simulink model "HBC_PHY_Layer"  (R2024a)
settings: Solver=FixedStepDiscrete  StartTime=0.0  StopTime=5E-2  RelTol=1e-3
values from neighbouring files (symbols this model uses):
  cfg = HBC_PHYFrameConfig(DataRate = '328Kbps', PilotInfo = '128', PSDULength = 254)    [MonteCarloSimulations.m]
libraries: hdlsllib x10, whdlio x1, commhdlcrc x1, commseqgen3 x1, vivadosimlib x1
settings Model: Creator=sookn  LastModifiedBy=sookn
settings OptimizationCC: BlockReduction=off  ConditionallyExecuteInputs=off  DefaultParameterBehavior=Inlined  OptimizeBlockIOStorage=off  EnhancedBackFolding=on  PassReuseOutputArgsAs=Individual arguments  OptimizeBlockOrder=speed  DifferentSizesBufferReuse=on  EfficientTunableParamExpr=on
settings DebuggingCC: SingleTaskRateTransMsg=error  ParameterTunabilityLossMsg=error
settings HardwareCC: ProdBitPerPointer=32  ProdBitPerSizeT=32  ProdBitPerPtrDiffT=32  ProdLargestAtomicFloat=None  ProdIntDivRoundTo=Undefined  ProdEndianess=Unspecified  ProdWordSize=32  ProdHWDeviceType=ASIC/FPGA->ASIC/FPGA  TargetBitPerPointer=64  TargetBitPerSizeT=64  TargetBitPerPtrDiffT=64  TargetLongLongMode=on  TargetIntDivRoundTo=Zero  TargetEndianess=LittleEndian  TargetWordSize=64  TargetHWDeviceType=Generic->Custom  ProdEqTarget=off
settings SFSimCC: MATLABDynamicMemAlloc=off
settings RTWCC: Description=SystemVerilog DPI Component Generator  SystemTargetFile=systemverilog_dpi_ert.tlc  TemplateMakefile=systemverilog_dpi_ert_default_tmf
settings CodeAppCC: ForceParamTrailComments=on  IgnoreCustomStorageClasses=off  MaxIdLength=256  OperatorAnnotations=on  SimulinkDataObjDesc=on  SFDataObjDesc=on  InsertBlockDesc=on
settings DPIERTTargetCC: TargetFcnLib=ansi_tfl_table_tmw.mat  GenFloatMathFcnCalls=NOT IN USE  TargetLangStandard=C99 (ISO)  CodeReplacementLibrary=None  UtilityFuncGeneration=Auto  MultiwordTypeDef=System defined  MultiwordLength=2048  DynamicStringBufferSize=256  GenerateFullHeader=on  InferredTypesCompatibility=off  GenerateSampleERTMain=off  GenerateTestInterfaces=off  ModelReferenceCompliant=on  ParMdlRefBuildCompliant=on  CompOptLevelCompliant=off  ConcurrentExecutionCompliant=off  IncludeMdlTerminateFcn=on  CombineOutputUpdateFcns=off  CombineSignalStateStructs=on  GroupInternalDataByFunction=off  SuppressErrorStatus=off  IncludeFileDelimiter=Auto  ERTCustomFileBanners=on  SupportAbsoluteTime=on  LogVarNameModifier=rt_  MatFileLogging=off  CodeInterfacePackaging=Reusable function  PurelyIntegerCode=off  SupportNonFinite=on  SupportComplex=on  SupportContinuousTime=on  SupportNonInlinedSFcns=on  RemoveDisableFunc=off  RemoveResetFunc=on  SupportVariableSizeSignals=off  ParenthesesLevel=Nominal  CastingMode=Nominal  MATLABClassNameForMDSCustomization=Simulink.SoftwareTarget.TargetSpecificTriggerConfigurationBase  ModelStepFunctionPrototypeControlCompliant=on  CPPClassGenCompliant=off  AutosarCompliant=off  MDXCompliant=off  GRTInterface=off  GenerateAllocFcn=on  UseToolchainInfoCompliant=on  GenerateSharedConstants=on  CoderGroups=[]  AccessMethods=[]  LookupTableObjectStructAxisOrder=1,2,3,4,...  LUTObjectStructOrderExplicitValues=Size,Breakpoints,Table  LUTObjectStructOrderEvenSpacing=Size,Breakpoints,Table  ArrayLayout=Column-major  UnsupportedSFcnMsg=error  ERTHeaderFileRootName=$R$E  ERTSourceFileRootName=$R$E  ERTDataFileRootName=$R_data  InstructionSetFMA=off  OptimizeReductions=off  LogToMDFFile=off  GenerateASAP2=off  DSAsUniqueAccess=off  ExtMode=off  ExtModeTransport=0  ExtModeStaticAlloc=off  ExtModeAutomaticAllocSize=on  ExtModeMaxTrigDuration=10  ExtModeStaticAllocSize=1000000  ExtModeTesting=off  ExtModeMexFile=ext_comm  ExtModeIntrfLevel=Level1  InlinedParameterPlacement=NonHierarchical  TargetOS=BareBoardExample  MultiInstanceErrorCode=Error  RootIOFormat=Part of model data structure  RTWCAPISignals=on  RTWCAPIParams=off  RTWCAPIStates=off  RTWCAPIRootIO=off  ERTSrcFileBannerTemplate=ert_code_template.cgt  ERTHdrFileBannerTemplate=ert_code_template.cgt  ERTDataSrcFileTemplate=ert_code_template.cgt  ERTDataHdrFileTemplate=ert_code_template.cgt  ERTCustomFileTemplate=example_file_process.tlc  EnableDataOwnership=off  SignalDisplayLevel=10  ParamTuneLevel=10  GlobalDataDefinition=Auto  DataDefinitionFile=global.c  GlobalDataReference=Auto  ERTFilePackagingFormat=Modular  RateTransitionBlockCode=Inline  DataReferenceFile=global.h  PreserveExpressionOrder=off  PreserveIfCondition=off  ConvertIfToSwitch=on  PreserveExternInFcnDecls=on  PreserveStaticInFcnDecls=on  SuppressUnreachableDefaultCases=on  EnableSignedLeftShifts=on  EnableSignedRightShifts=on  ImplementImageWithCVMat=off  IndentStyle=K&R  IndentSize=2  NewlineStyle=Default  MaxLineWidth=80  EnableUserReplacementTypes=off  MaxIdInt64=MAX_int64_T  MinIdInt64=MIN_int64_T  MaxIdUint64=MAX_uint64_T  MaxIdInt32=MAX_int32_T  MinIdInt32=MIN_int32_T  MaxIdUint32=MAX_uint32_T  MaxIdInt16=MAX_int16_T  MinIdInt16=MIN_int16_T  MaxIdUint16=MAX_uint16_T  MaxIdInt8=MAX_int8_T  MinIdInt8=MIN_int8_T  MaxIdUint8=MAX_uint8_T  BooleanTrueId=true  BooleanFalseId=false  MemSecPackage=--- None ---  MemSecDataConstants=Default  MemSecDataIO=Default  MemSecDataInternal=Default  MemSecDataParameters=Default  MemSecFuncInitTerm=Default  MemSecFuncExecute=Default  MemSecFuncSharedUtil=Default  GroupConstants=Default  GroupRootInputs=Default  GroupRootOutputs=Default  GroupInternal=Default  GroupParameters=Default  GroupDataTransfer=Default  GroupSharedLocalDataStores=Default  GroupInstanceSpecificParameters=Default  GroupModelData=Default  ArrayContainerType=C-style array  DPICustomizeSystemVerilogCode=off  DPISystemVerilogTemplate=svdpi_event.vgt  DPIReportRunTimeError=off  DPIScalarizePorts=off  DPIRunTimeErrorSeverity=Fatal  DPIGenerateTestBench=off  DPITestBenchSimulator=Mentor Graphics Questasim  DPITestPointAccessFcnInterface=None  DPIFixedPointDataType=CompatibleCType  DPIPortConnection=Port list  DPICompositeDataType=Flattened  DPIComponentTemplateType=Sequential

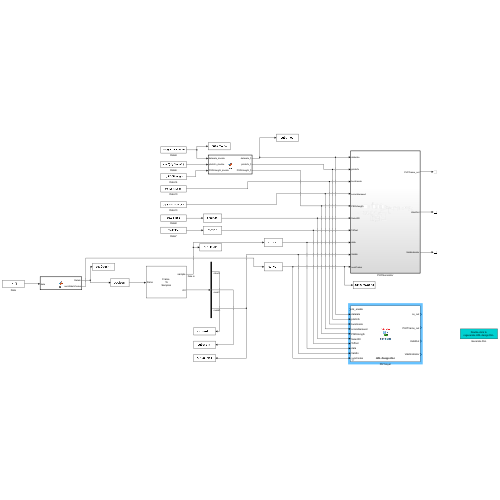
[thumbnail: Simulink's stored preview of the top-level diagram]
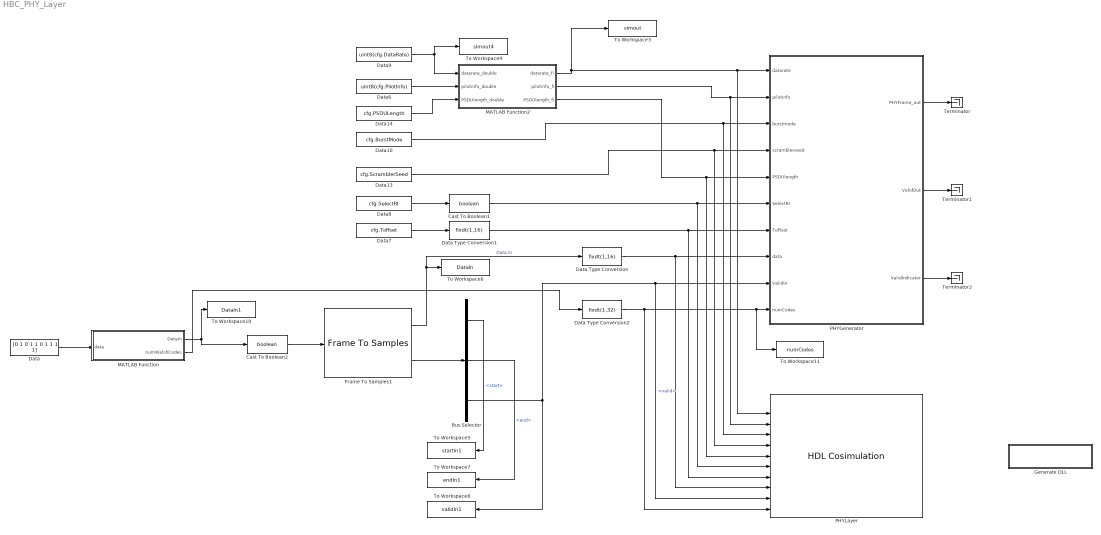
== system HBC_PHY_Layer ==
  Bus Selector : BusSelector  OutputSignals=start,end,valid
  Cast To Boolean1 : DataTypeConversion  OutDataTypeStr=boolean  SaturateOnIntegerOverflow=off  RndMeth=Floor
  Cast To Boolean2 : DataTypeConversion  OutDataTypeStr=boolean  SaturateOnIntegerOverflow=off  RndMeth=Floor
  Data : Constant  Value=[0 1 0 1 1 0 1 1 1 1]  SampleTime=-1
  Data Type Conversion : DataTypeConversion  OutMax=[1]  OutDataTypeStr=fixdt(1,16)  SaturateOnIntegerOverflow=off  RndMeth=Floor
  Data Type Conversion1 : DataTypeConversion  OutMax=[16]  OutDataTypeStr=fixdt(1,16)  SaturateOnIntegerOverflow=off  RndMeth=Floor
  Data Type Conversion2 : DataTypeConversion  OutMax=[32]  OutDataTypeStr=fixdt(1,32)  SaturateOnIntegerOverflow=off  RndMeth=Floor
  Data10 : Constant  Value=cfg.BurstMode  SampleTime=(9056*8)/(42E6)
  Data13 : Constant  Value=cfg.ScramblerSeed  SampleTime=(9056*8)/(42E6)
  Data14 : Constant  Value=cfg.PSDULength  SampleTime=-1
  Data6 : Constant  Value=uint8(cfg.PilotInfo)  SampleTime=-1
  Data7 : Constant  Value=cfg.Toffset  SampleTime=(9056*8)/(42E6)
  Data8 : Constant  Value=cfg.SelectRI  SampleTime=(9056*8)/(42E6)
  Data9 : Constant  Value=uint8(cfg.DataRate)  SampleTime=-1
  Frame To Samples1 : whdlio/Frame To Samples  InterSampleIdleCycles=0  InterFrameIdleCycles=4  OutputSize=1  InterleaveSamples=off
  Generate DLL : Subsystem
      settings: OpenFcn=eval('hdlverifier_gendll_PHYLayer');
      mask Display: disp(['Double-click to' char(10) 'regenerate HDL design DLL'])
  MATLAB Function : MATLAB Function  TreatAsAtomicUnit=on
  MATLAB Function2 : MATLAB Function  TreatAsAtomicUnit=on
  PHYGenerator : Subsystem  TreatAsAtomicUnit=on
  PHYLayer : vivadosimlib/HDL Cosimulation  PortPaths=/PHYLayer/clk_enable;/PHYLayer/datarate;/PHYLayer/pilotinfo;/PHYLayer/burstmode;/PHYLayer/scramblerseed;/PHYLayer/PSDUlength;/PHYLayer/SelectRI;/PHYLayer/Toffset;/PHYLayer/data;/PHYLayer/ValidIn;/PHYLayer/numCodes;/PHYLayer/ce_out;/PHYLayer/PHYFrame_out;/PHYLayer/ValidOut;/PHYLayer/ValidIndicator;  PortModes=[1 1 1 1 1 1 1 1 1 1 1 2 2 2 2 ]  PortTimes=[-1,-1,-1,-1,-1,-1,-1,-1,-1,-1,-1,1,1,1,1]  PortSigns=[-1,-1,-1,-1,-1,-1,-1,-1,-1,-1,-1,-1,-1,-1,-1,]  PortFracLengths=[0,0,0,0,0,0,0,0,0,0,0,0,0,0,0]  PortWordLengths=[-1,-1,-1,-1,-1,-1,-1,-1,-1,-1,-1,1,1,1,1]  PortHDLWordSizes=[1,3,3,1,1,9,1,16,16,1,32,1,1,1,1]  CommLocal=on  CommSharedMemory=off  CommPortNumber=0  CommShowInfo=on  ClockPaths=/PHYLayer/clk;/PHYLayer/reset;  ClockModes=[2 3 ]  ClockTimes=[1e-08 8e-09 ]  TimingMode=s  TimingScaleFactor=1  idxCellArray={'UNUSED_VAR'}  CosimBypass=Full Simulation  AllowDirectFeedthrough=on  ProductName=EDA Simulator Link VS  RunAutoTimescale=on  HdlClocks=/PHYLayer/clk 10 ns;  PreRunTime=10  PreRunTimeUnit=ns
  Terminator : Terminator
  Terminator1 : Terminator
  Terminator2 : Terminator
  To Workspace10 : ToWorkspace  VariableName=DataIn1  SaveFormat=Structure With Time  SampleTime=-1
  To Workspace11 : ToWorkspace  VariableName=numCodes  SaveFormat=Structure With Time  SampleTime=-1
  To Workspace3 : ToWorkspace  VariableName=simout  SaveFormat=Structure With Time  SampleTime=-1
  To Workspace4 : ToWorkspace  VariableName=simout4  SaveFormat=Structure With Time  SampleTime=-1
  To Workspace5 : ToWorkspace  VariableName=startIn1  SaveFormat=Structure With Time  SampleTime=-1
  To Workspace6 : ToWorkspace  VariableName=DataIn  SaveFormat=Structure With Time  SampleTime=-1
  To Workspace7 : ToWorkspace  VariableName=endIn1  SaveFormat=Structure With Time  SampleTime=-1
  To Workspace8 : ToWorkspace  VariableName=validIn1  SaveFormat=Structure With Time  SampleTime=-1
  wires:
  Cast To Boolean2/1 -> Frame To Samples1/1
  Data9/1 -> MATLAB Function2/1(datarate_double), To Workspace4/1
  Data14/1 -> MATLAB Function2/3(PSDUlength_double)
  Frame To Samples1/1 -> Data Type Conversion/1, To Workspace6/1  "Data In"
  Data13/1 -> PHYLayer/5, PHYGenerator/4(scramblerseed)
  Data8/1 -> Cast To Boolean1/1
  Data Type Conversion1/1 -> PHYLayer/8, PHYGenerator/7(Toffset)
  MATLAB Function2/2(pilotinfo_fi) -> PHYLayer/3, PHYGenerator/2(pilotinfo)
  MATLAB Function/2(numWalshCodes) -> Data Type Conversion2/1
  Frame To Samples1/2 -> Bus Selector/1
  Data Type Conversion2/1 -> PHYLayer/11, To Workspace11/1, PHYGenerator/10(numCodes)
  Data6/1 -> MATLAB Function2/2(pilotinfo_double)
  Bus Selector/3 -> PHYLayer/10, PHYGenerator/9(ValidIn), To Workspace8/1  "<valid>"
  MATLAB Function2/3(PSDUlength_fi) -> PHYLayer/6, PHYGenerator/5(PSDUlength)
  PHYGenerator/1(PHYFrame_out) -> Terminator/1
  Bus Selector/2 -> To Workspace7/1  "<end>"
  MATLAB Function/1(DataIn) -> Cast To Boolean2/1, To Workspace10/1
  PHYGenerator/2(ValidOut) -> Terminator1/1
  Cast To Boolean1/1 -> PHYLayer/7, PHYGenerator/6(SelectRI)
  Bus Selector/1 -> To Workspace5/1  "<start>"
  Data/1 -> MATLAB Function/1(data)
  Data7/1 -> Data Type Conversion1/1
  MATLAB Function2/1(datarate_fi) -> To Workspace3/1, PHYLayer/2, PHYGenerator/1(datarate)
  Data10/1 -> PHYLayer/4, PHYGenerator/3(burstmode)
  PHYGenerator/3(ValidIndicator) -> Terminator2/1
  Data Type Conversion/1 -> PHYLayer/9, PHYGenerator/8(data)

== system HBC_PHY_Layer/Generate DLL ==

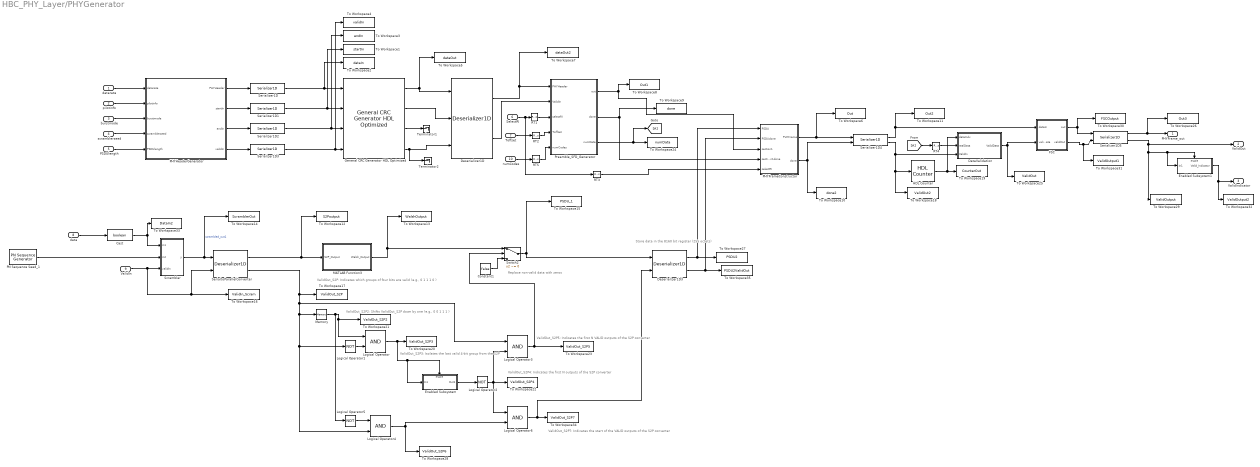
== system HBC_PHY_Layer/PHYGenerator ==
  note: Replace non-valid data with zeros
  note: ValidOut_S2P: Indicates which groups of four bits are valid (e.g., 0 1 1 1 0 )
  note: ValidOut_S2P2: Shifts ValidOut_S2P down by one (e.g., 0 0 1 1 1 )
  note: ValidOut_S2P3: Isolates the last valid 4-bit group from the S2P
  note: ValidOut_S2P4: Indicates the first N outputs of the S2P converter
  note: ValidOut_S2P5: Indicates the first N VALID outputs of the S2P converter
  note: ValidOut_S2P7: Indicates the start of the VALID outputs of the S2P converter
  note: Store data in the 8160 bit register (255 octets)
  datarate : Inport
  pilotinfo : Inport  Port=2
  burstmode : Inport  Port=3
  scramblerseed : Inport  Port=4
  PSDUlength : Inport  Port=5
  SelectRI : Inport  Port=6
  Toffset : Inport  Port=7
  data : Inport  Port=8
  ValidIn : Inport  Port=9
  numCodes : Inport  Port=10
  Cast : DataTypeConversion  OutDataTypeStr=boolean  SaturateOnIntegerOverflow=off  RndMeth=Floor
  Constant1 : Constant  Value=false  SampleTime=-1
  DataValidation : MATLAB Function  TreatAsAtomicUnit=on
  Deserializer1D : hdlsllib/HDL Operations/Deserializer1D  Ratio=4  IdleCycles=0  InitialCondition=0  startIn=on  validIn=on  validOut=on  inputDataDimensions=-1  inputSampleTime=-1  inputSignalType=auto
  Deserializer1D3 : hdlsllib/HDL Operations/Deserializer1D  Ratio=510  IdleCycles=0  InitialCondition=0  startIn=on  validIn=off  validOut=on  inputDataDimensions=-1  inputSampleTime=-1  inputSignalType=auto
  Enabled Subsystem : Subsystem  TreatAsAtomicUnit=on
  Enabled Subsystem1 : Subsystem  TreatAsAtomicUnit=on
  FSC : MATLAB Function  TreatAsAtomicUnit=on
  From : From
  General CRC Generator HDL Optimized : commhdlcrc/General CRC Generator HDL Optimized  Polynomial=[1, 1, 0, 0, 0, 1, 1, 0, 1]  InitialState=0  DirectMethod=off  ReflectInput=off  ReflectCRCChecksum=off  FinalXORValue=0  SimulateUsing=Code generation
  Goto : Goto
  HDL Counter : hdlsllib/Sources/HDL Counter  CountType=Count limited  CountInit=1  CountStep=1  CountMax=9056  CountFromType=Initial value  CountFrom=1  CountResetPort=off  CountLoadPort=off  CountEnbPort=on  CountDirPort=off  CountHitOutputPort=off  CountDataType=Unsigned  CountWordLen=14  CountFracLen=0  CountSampTime=1
  Logical Operator{,3..4,6} (4 alike) : Logic  IconShape=distinctive  AllPortsSameDT=off  OutDataTypeStr=boolean
  Logical Operator1 : Logic  Operator=NOT  IconShape=distinctive  AllPortsSameDT=off  OutDataTypeStr=boolean
  Logical Operator2 : Logic  Operator=NOT  IconShape=distinctive  AllPortsSameDT=off  OutDataTypeStr=boolean
  Logical Operator5 : Logic  Operator=NOT  IconShape=distinctive  AllPortsSameDT=off  OutDataTypeStr=boolean
  MATLAB Function3 : MATLAB Function  TreatAsAtomicUnit=on
  Memory : Memory  InheritSampleTime=on
  PHYFrameConstructor : MATLAB Function  TreatAsAtomicUnit=on
  PHYHeaderGenerator : MATLAB Function  TreatAsAtomicUnit=on
  PN Sequence Seed_1 : commseqgen3/PN Sequence Generator  poly='z32 + z21 + z1 + 1'  ini_sta=[1 0 0 0 1 0 1 0 0 1 0 1 1 1 1 1 0 1 1 0 0 0 1 0 0 0 0 1 1 1 1 1]  outBitMaskSource=Dialog parameter  shift=0  outVarSiz=off  maxOutSizeMode=Dialog parameter  maxOutSize=[10 1]  Ts=(9056*8)/(4*510*(42E6))  sampPerFrame=1  reset=off  bitPackedOutputs=off  outDataType=boolean  numPackedBits=8  bitPackDataSigned=off  bitPackedOutDType=double
      settings: LibrarySourceBlock=|
      | commhdlsource/PN Sequence
      | Generator
  Preamble_SFD_Generator : MATLAB Function  TreatAsAtomicUnit=on
  RT{1..3,5} (4 alike) : RateTransition  Integrity=off  OutPortSampleTime=(9056*8)/(42E6)
  RT4 : RateTransition  Integrity=off  OutPortSampleTime=8/(42E6)
  Scrambler : MATLAB Function  TreatAsAtomicUnit=on
  Serializer1D{,1..3} (4 alike) : hdlsllib/HDL Operations/Serializer1D  Ratio=4  IdleCycles=0  validIn=off  startOut=off  validOut=off  inputDataDimensions=-1  inputSampleTime=-1  inputSignalType=auto
  Serializer1D4 : hdlsllib/HDL Operations/Serializer1D  Ratio=9056  IdleCycles=0  validIn=on  startOut=off  validOut=on  inputDataDimensions=-1  inputSampleTime=-1  inputSignalType=auto
  Serializer1D5 : hdlsllib/HDL Operations/Serializer1D  Ratio=8  IdleCycles=0  validIn=on  startOut=off  validOut=on  inputDataDimensions=-1  inputSampleTime=-1  inputSignalType=auto
  SerialtoParallelConverter : hdlsllib/HDL Operations/Deserializer1D  Ratio=4  IdleCycles=0  InitialCondition=0  startIn=off  validIn=on  validOut=on  inputDataDimensions=-1  inputSampleTime=-1  inputSignalType=auto
  Switch2 : Switch  Criteria=u2 ~= 0  SaturateOnIntegerOverflow=off  InputSameDT=off
  Terminator1 : Terminator
  Terminator2 : Terminator
  To Workspace1 : ToWorkspace  VariableName=startIn  SaveFormat=Structure With Time  SampleTime=-1
  To Workspace10 : ToWorkspace  VariableName=done2  SaveFormat=Structure With Time  SampleTime=-1
  To Workspace11 : ToWorkspace  VariableName=Out2  SaveFormat=Structure With Time  SampleTime=-1
  To Workspace12 : ToWorkspace  VariableName=S2Poutput  SaveFormat=Structure With Time  SampleTime=-1
  To Workspace13 : ToWorkspace  VariableName=WalshOutput  SaveFormat=Structure With Time  SampleTime=-1
  To Workspace14 : ToWorkspace  VariableName=ScramblerOut  SaveFormat=Structure With Time  SampleTime=-1
  To Workspace15 : ToWorkspace  VariableName=PSDU_1  SaveFormat=Structure With Time  SampleTime=-1
  To Workspace16 : ToWorkspace  VariableName=ValidIn_Scram  SaveFormat=Structure With Time  SampleTime=-1
  To Workspace17 : ToWorkspace  VariableName=ValidOut_S2P  SaveFormat=Structure With Time  SampleTime=-1
  To Workspace18 : ToWorkspace  VariableName=ValidOut2  SaveFormat=Structure With Time  SampleTime=-1
  To Workspace19 : ToWorkspace  VariableName=CounterOut  SaveFormat=Structure With Time  SampleTime=-1
  To Workspace2 : ToWorkspace  VariableName=dataIn  SaveFormat=Structure With Time  SampleTime=-1
  To Workspace20 : ToWorkspace  VariableName=ValidOut_S2P3  SaveFormat=Structure With Time  SampleTime=-1
  To Workspace21 : ToWorkspace  VariableName=ValidOut_S2P2  SaveFormat=Structure With Time  SampleTime=-1
  To Workspace22 : ToWorkspace  VariableName=ValidOut_S2P4  SaveFormat=Structure With Time  SampleTime=-1
  To Workspace23 : ToWorkspace  VariableName=ValidOut_S2P5  SaveFormat=Structure With Time  SampleTime=-1
  To Workspace24 : ToWorkspace  VariableName=numData  SaveFormat=Structure With Time  SampleTime=-1
  To Workspace25 : ToWorkspace  VariableName=ValidOut  SaveFormat=Structure With Time  SampleTime=-1
  To Workspace26 : ToWorkspace  VariableName=Out3  SaveFormat=Structure With Time  SampleTime=-1
  To Workspace27 : ToWorkspace  VariableName=PSDU2  SaveFormat=Structure With Time  SampleTime=-1
  To Workspace28 : ToWorkspace  VariableName=ValidOut_S2P6  SaveFormat=Structure With Time  SampleTime=-1
  To Workspace29 : ToWorkspace  VariableName=ValidOutput  SaveFormat=Structure With Time  SampleTime=-1
  To Workspace3 : ToWorkspace  VariableName=endIn  SaveFormat=Structure With Time  SampleTime=-1
  To Workspace30 : ToWorkspace  VariableName=FSCOutput  SaveFormat=Structure With Time  SampleTime=-1
  To Workspace31 : ToWorkspace  VariableName=ValidOutput1  SaveFormat=Structure With Time  SampleTime=-1
  To Workspace32 : ToWorkspace  VariableName=ValidOutput2  SaveFormat=Structure With Time  SampleTime=-1
  To Workspace33 : ToWorkspace  VariableName=DataIn2  SaveFormat=Structure With Time  SampleTime=-1
  To Workspace34 : ToWorkspace  VariableName=ValidOut_S2P7  SaveFormat=Structure With Time  SampleTime=-1
  To Workspace35 : ToWorkspace  VariableName=PSDU2ValidOut  SaveFormat=Structure With Time  SampleTime=-1
  To Workspace4 : ToWorkspace  VariableName=validIn  SaveFormat=Structure With Time  SampleTime=-1
  To Workspace5 : ToWorkspace  VariableName=dataOut  SaveFormat=Structure With Time  SampleTime=-1
  To Workspace6 : ToWorkspace  VariableName=Out  SaveFormat=Structure With Time  SampleTime=-1
  To Workspace7 : ToWorkspace  VariableName=dataOut2  SaveFormat=Structure With Time  SampleTime=-1
  To Workspace8 : ToWorkspace  VariableName=Out1  SaveFormat=Structure With Time  SampleTime=-1
  To Workspace9 : ToWorkspace  VariableName=done  SaveFormat=Structure With Time  SampleTime=-1
  PHYFrame_out : Outport  VectorParamsAs1DForOutWhenUnconnected=off
  ValidOut : Outport  Port=2  VectorParamsAs1DForOutWhenUnconnected=off
  ValidIndicator : Outport  Port=3  VectorParamsAs1DForOutWhenUnconnected=off
  wires:
  scramblerseed/1 -> PHYHeaderGenerator/4(scramblerseed)
  datarate/1 -> PHYHeaderGenerator/1(datarate)
  burstmode/1 -> PHYHeaderGenerator/3(burstmode)
  PSDUlength/1 -> PHYHeaderGenerator/5(PSDUlength)
  PHYHeaderGenerator/1(PHYHeader) -> Serializer1D/1
  pilotinfo/1 -> PHYHeaderGenerator/2(pilotinfo)
  Serializer1D/1 -> To Workspace2/1, General CRC Generator HDL Optimized/1
  PHYHeaderGenerator/2(startIn) -> Serializer1D1/1
  PHYHeaderGenerator/3(endIn) -> Serializer1D2/1
  PHYHeaderGenerator/4(validIn) -> Serializer1D3/1
  Serializer1D1/1 -> To Workspace1/1, General CRC Generator HDL Optimized/2
  Serializer1D2/1 -> To Workspace3/1, General CRC Generator HDL Optimized/3
  Serializer1D3/1 -> To Workspace4/1, General CRC Generator HDL Optimized/4
  General CRC Generator HDL Optimized/1 -> Deserializer1D/1, To Workspace5/1
  General CRC Generator HDL Optimized/2 -> Deserializer1D/2
  General CRC Generator HDL Optimized/3 -> Terminator1/1
  General CRC Generator HDL Optimized/4 -> Deserializer1D/3, Terminator2/1
  Deserializer1D/1 -> To Workspace7/1, Preamble_SFD_Generator/1(PHYHeader)
  Deserializer1D/2 -> Preamble_SFD_Generator/2(ValidIn)
  Toffset/1 -> RT2/1
  Preamble_SFD_Generator/1(out) -> PHYFrameConstructor/3(section1), To Workspace8/1
  Preamble_SFD_Generator/2(done) -> PHYFrameConstructor/4(section1done), To Workspace9/1
  MATLAB Function3/1(Walsh_Output) -> Switch2/1, To Workspace13/1
  Constant1/1 -> Switch2/3
  ValidIn/1 -> To Workspace16/1, SerialtoParallelConverter/2, Scrambler/3(validIn)
  SerialtoParallelConverter/2 -> Logical Operator4/2, Logical Operator1/1, Memory/1, Logical Operator3/1, To Workspace17/1
  PN Sequence Seed_1/1 -> Scrambler/2(in2)
  SerialtoParallelConverter/1 -> To Workspace12/1, MATLAB Function3/1(S2P_Output)
  Scrambler/1(y) -> To Workspace14/1, SerialtoParallelConverter/1  "scrambled_out1"
  Memory/1 -> Logical Operator5/1, Logical Operator/1, To Workspace21/1
  Logical Operator1/1 -> Logical Operator/2
  Logical Operator/1 -> Enabled Subsystem/1(In1), Enabled Subsystem/Enable, To Workspace20/1
  Enabled Subsystem/1(Out1) -> Logical Operator2/1
  Logical Operator2/1 -> Logical Operator6/1, Logical Operator3/2, To Workspace22/1
  Logical Operator3/1 -> To Workspace23/1, Switch2/2
  Logical Operator4/1 -> To Workspace28/1, Logical Operator6/2
  Logical Operator5/1 -> Logical Operator4/1
  Logical Operator6/1 -> Deserializer1D3/2, To Workspace34/1
  Switch2/1 -> Deserializer1D3/1, To Workspace15/1
  SelectRI/1 -> RT3/1, RT1/1
  numCodes/1 -> RT5/1
  Deserializer1D3/1 -> PHYFrameConstructor/1(PSDU), To Workspace27/1
  Deserializer1D3/2 -> PHYFrameConstructor/2(PSDUdone), To Workspace35/1
  RT1/1 -> Preamble_SFD_Generator/3(selectRI)
  RT2/1 -> Preamble_SFD_Generator/4(Toffset)
  PHYFrameConstructor/1(PHYFrame) -> To Workspace6/1, Serializer1D4/1
  PHYFrameConstructor/2(done) -> To Workspace10/1, Serializer1D4/2
  RT3/1 -> PHYFrameConstructor/5(selectRI)
  Serializer1D4/1 -> To Workspace11/1, FSC/1(dataIn)
  HDL Counter/1 -> DataValidation/1(dataIndx), To Workspace19/1
  Serializer1D4/2 -> DataValidation/3(ValidIn), HDL Counter/1, To Workspace18/1
  RT5/1 -> Preamble_SFD_Generator/5(numCodes)
  Preamble_SFD_Generator/3(numData) -> Goto/1, To Workspace24/1
  From/1 -> RT4/1
  DataValidation/1(ValidData) -> To Workspace25/1, FSC/2(validData)
  RT4/1 -> DataValidation/2(realData)
  FSC/1(out) -> Serializer1D5/1, To Workspace30/1
  Serializer1D5/1 -> PHYFrame_out/1, To Workspace26/1
  Serializer1D5/2 -> ValidOut/1, Enabled Subsystem1/1(In1), Enabled Subsystem1/Enable, To Workspace29/1
  FSC/2(validOut) -> To Workspace31/1, Serializer1D5/2
  Enabled Subsystem1/1(Valid_Indicator) -> ValidIndicator/1, To Workspace32/1
  data/1 -> Cast/1
  Cast/1 -> To Workspace33/1, Scrambler/1(in1)

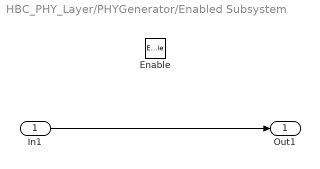
== system HBC_PHY_Layer/PHYGenerator/Enabled Subsystem ==
  In1 : Inport
  Enable : EnablePort
  Out1 : Outport
  wires:
  In1/1 -> Out1/1

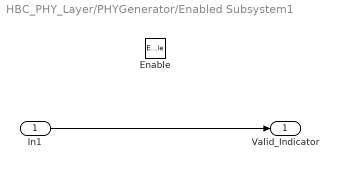
== system HBC_PHY_Layer/PHYGenerator/Enabled Subsystem1 ==
  In1 : Inport
  Enable : EnablePort
  Valid_Indicator : Outport
  wires:
  In1/1 -> Valid_Indicator/1

== matlab function HBC_PHY_Layer/PHYGenerator/FSC ==
  data: dataIn input; out output; validData input; validOut output
function [out, validOut] = FSC(dataIn, validData)
%#codegen
out = boolean(zeros(1,8)); 
FSC1 = boolean([0 1 0 1 0 1 0 1]); 
FSC0 = boolean([1 0 1 0 1 0 1 0]); 
validOut = false; 

if (validData)
    if (dataIn) % Bit is a logic '1'
        out = FSC1; 
    else % Bit is a logic '0'
        out = FSC0; 
    end
    validOut = true; 
end

== matlab function HBC_PHY_Layer/MATLAB Function2 ==
  data: datarate_double input; datarate_fi output; pilotinfo_double input; pilotinfo_fi output; PSDUlength_double input; PSDUlength_fi output
function [datarate_fi, pilotinfo_fi, PSDUlength_fi] = fcn(datarate_double, pilotinfo_double, PSDUlength_double)
datarate_sum = sum(datarate_double);
pilotinfo_sum = sum(pilotinfo_double); 

datarate_fi = fi(0,0,3,0);
pilotinfo_fi = fi(0,0,3,0);
PSDUlength_fi = fi(PSDUlength_double,0,9,0);
% , pilotinfo, burstmode, scramblerseed, PSDUlength

% Data rate
switch datarate_sum
    case sum(double('164Kbps'))
        datarate_fi = fi(1,0,3,0);
    case sum(double('328Kbps'))
        datarate_fi = fi(2,0,3,0);
    case sum(double('656Kbps'))
        datarate_fi = fi(3,0,3,0);
    case sum(double('1.3125Mbps'))
        datarate_fi = fi(4,0,3,0);
    case sum(double('RI'))
        datarate_fi = fi(5,0,3,0);
    case sum(double('Reserved'))
        datarate_fi = fi(6,0,3,0);
end 

% Pilot Info
switch pilotinfo_sum
    case sum(double('64'))
        pilotinfo_fi = fi(1,0,3,0);
    case sum(double('128'))
        pilotinfo_fi = fi(2,0,3,0);
    case sum(double('Reserved'))
        pilotinfo_fi = fi(3,0,3,0);
    case sum(double('NA')) % No insertion
        pilotinfo_fi = fi(4,0,3,0);
end

== matlab function HBC_PHY_Layer/PHYGenerator/PHYHeaderGenerator ==
  data: datarate input; PHYHeader output; pilotinfo input; burstmode input; scramblerseed input; PSDUlength input; startIn output; endIn output; validIn output
function [PHYHeader, startIn, endIn, validIn]  = fcn(datarate, pilotinfo, burstmode, scramblerseed, PSDUlength)

% persistent CRC_IEEE802_15_6_gen;
% if isempty(CRC_IEEE802_15_6_gen)
%     CRC_IEEE802_15_6_gen = comm.HDLCRCGenerator('Polynomial', [1 1 0 0 0 1 1 0 1]);
% end

PHYHeader = boolean(zeros(32,1)); 
data = boolean(zeros(1,32));

% , pilotinfo, burstmode, scramblerseed, PSDUlength
message = boolean(zeros(1,24)); 
PSDUlength_int = int32(PSDUlength);
PSDUlength_bin = boolean(zeros(1,8)); 
rem = 0; 

%PSDUlength_bin = boolean(zeros(1,8));

% Data rate
switch datarate
    case fi(1)
        message(1:3) = boolean([0 0 0]);
    case fi(2)
        message(1:3) = boolean([0 0 1]);
    case fi(3)
        message(1:3) = boolean([0 1 0]);
    case fi(4)
        message(1:3) = boolean([0 1 1]);
    case fi(5)
        message(1:3) = boolean([1 1 1]);
    case fi(6)
        message(1:3) = boolean([1 0 0]);
end 

% Pilot Info
switch pilotinfo
    case fi(1)
        message(4:6) = boolean([0 1 0]);
    case fi(2)
        message(4:6) = boolean([0 1 1]);
    case fi(3)
        message(4:6) = boolean([0 0 0]);
    case fi(4) % No insertion
        message(4:6) = boolean([1 1 0]);
end 


% Bits 7-8 reserved

% Burst Mode (bit-9)
switch burstmode
    case true
        message(9) = true;
    case false
        message(9) = false;
end
 
% Bits 10-11 Reserved

% Scrambler Seed (bit-12)
switch scramblerseed
    case true
        message(12) = true;
        %scramblerseed = boolean([1 0 0 0 1 0 1 0 0 1 0 1 1 1 1 1 0 1 1 0 0 0 1 0 0 0 0 1 1 1 1 1]); 
    case false
        message(12) = false;
        %scramblerseed = [0 1 1 0 1 0 0 1 0 1 0 1 0 1 0 0 0 0 0 0 0 0 0 1 0 1 0 1 0 0 1 0]; 
end
 
% Bits 13-16 Reserved

% PSDU Length (17-24)
num = PSDUlength_int;
powers = [int32(128) int32(64) int32(32) int32(16) int32(8) int32(4) int32(2) int32(1)];
for i=1:1:8
    if (num >= powers(i))
        PSDUlength_bin(i) = true; 
    else 
        PSDUlength_bin(i) = false;
    end
    num = num - powers(i); 

message(17:24) = PSDUlength_bin(1:8);
data(1:24) = message(1:24);
PHYHeader = data';

% CRC Generation

dataIn_width = 8;
%mlen = length(PHYHeader)/dataIn_width;
dlen = length(message)/dataIn_width; 
startIn = boolean([1, zeros(1,dlen)])';
endIn = boolean([zeros(1,dlen-1), 1, 0])';
validIn = boolean([ones(1,dlen), 0])';


end

== matlab function HBC_PHY_Layer/PHYGenerator/Preamble_SFD_Generator ==
  data: PHYHeader input; out output; ValidIn input; done output; selectRI input; Toffset input; numCodes input; numData output
function [out, done, numData] = fcn(PHYHeader, ValidIn, selectRI, Toffset, numCodes)

%Toffset = double(toffset);
%out0 = boolean(zeros(1,800));

out = boolean(zeros(1,896)); % Output register
done = false; % Done indication
numData = int32(0); % Represents the number of valid bits that require FSC coding
%done1 = false; 

if(ValidIn) % The PHYHeader has been successfully generated

    % -------------------- Preamble ------------------------------------------

    rep4_preamble_goldseq = boolean(zeros(1,256));
    %rep8_preamble_goldseq = boolean(zeros(256,8));
    preamble_goldseq = boolean([1 1 0 0 0 1 0 0 1 1 0 0 1 0 1 0 ...
        0 1 0 1 0 0 0 0 0 0 0 1 1 0 0 0 ...
        1 1 1 1 1 0 1 0 1 1 1 0 0 1 0 0 ...
        1 0 1 1 1 0 0 1 1 0 0 0 0 0 1 0]);
    rep4_preamble_goldseq = repmat(preamble_goldseq, 1, 4);

    % --------------------- SFD ----------------------------------------------

    SFD_goldseq = boolean([0 1 0 1 0 1 1 0 0 1 0 1 1 1 0 1 ...
        1 1 0 1 1 0 1 1 1 1 0 0 1 0 1 0 ...
        0 1 0 1 1 0 0 0 0 0 1 0 0 1 1 0 ...
        0 1 1 1 1 0 1 0 1 1 0 0 1 1 0 1]);
    rep8_SFD_RI_0 = boolean(zeros(1,512));
    rep8_SFD_RI_1 = boolean(zeros(1,608));
    % preamble_SFD0 = boolean(zeros(1,768));
    % preamble_SFD1 = boolean(zeros(1,864));

    SFD_RI_1 = boolean(zeros(1,76));
    % Select RI Multiplexing functionality
    switch selectRI
        case 0
            rep8_SFD_RI_0 = repmat(SFD_goldseq, 1, 8);
            out(1:800) = [rep4_preamble_goldseq, rep8_SFD_RI_0, PHYHeader']; % Preamble and RI = 0 SFD code
            numData = 800 + int32(16*numCodes); % 800 + N-groups of 16 bits.
            done = true;
        case 1
            if Toffset == fi(1)
                SFD_RI_1 = [SFD_goldseq, boolean(zeros(1,12))];
            elseif Toffset == fi(2)
                SFD_RI_1 = [boolean(zeros(1,2)), SFD_goldseq, boolean(zeros(1,10))];
            elseif Toffset == fi(3)
                SFD_RI_1 = [boolean(zeros(1,4)), SFD_goldseq, boolean(zeros(1,8))];
            elseif Toffset == fi(4)
                SFD_RI_1 = [boolean(zeros(1,6)), SFD_goldseq, boolean(zeros(1,6))];
            elseif Toffset == fi(5)
                SFD_RI_1 = [boolean(zeros(1,8)), SFD_goldseq, boolean(zeros(1,4))];
            else
                SFD_RI_1 = [SFD_goldseq, boolean(zeros(1,12))];
            end
            rep8_SFD_RI_1 = repmat(SFD_RI_1,1,8);
            out = [rep4_preamble_goldseq, rep8_SFD_RI_1, PHYHeader']; % Preamble and RI = 1 SFD code
            numData = 896 + int32(16*numCodes); % 896 + N-groups of 16 bits.
            done = true;
    end
end
end

== matlab function HBC_PHY_Layer/PHYGenerator/Scrambler ==
  data: in1 input; y output; in2 input; validIn input
function y = XOR(in1, in2, validIn)
%#codegen
y = false;
if validIn
    y = xor(in1,in2);  
end

== matlab function HBC_PHY_Layer/PHYGenerator/MATLAB Function3 ==
  data: S2P_Output input; Walsh_Output output
function Walsh_Output = WalshCoding(S2P_Output)

Walsh_Output = boolean(zeros(1,16)); 
S2P_Output_dec = S2P_Output(4)*(8) + S2P_Output(3)*(4) + S2P_Output(2)*(2) + S2P_Output(1)*(1); 

WALSH16_CODES = boolean([1 1 1 1 1 1 1 1 1 1 1 1 1 1 1 1; 
                 1 0 1 0 1 0 1 0 1 0 1 0 1 0 1 0; 
                 1 1 0 0 1 1 0 0 1 1 0 0 1 1 0 0; 
                 1 0 0 1 1 0 0 1 1 0 0 1 1 0 0 1;
                 1 1 1 1 0 0 0 0 1 1 1 1 0 0 0 0; 
                 1 0 1 0 0 1 0 1 1 0 1 0 0 1 0 1;
                 1 1 0 0 0 0 1 1 1 1 0 0 0 0 1 1;
                 1 0 0 1 0 1 1 0 1 0 0 1 0 1 1 0;
                 1 1 1 1 1 1 1 1 0 0 0 0 0 0 0 0;
                 1 0 1 0 1 0 1 0 0 1 0 1 0 1 0 1;
                 1 1 0 0 1 1 0 0 0 0 1 1 0 0 1 1;
                 1 0 0 1 1 0 0 1 0 1 1 0 0 1 1 0;
                 1 1 1 1 0 0 0 0 0 0 0 0 1 1 1 1;
                 1 0 1 0 0 1 0 1 0 1 0 1 1 0 1 0;
                 1 1 0 0 0 0 1 1 0 0 1 1 1 1 0 0;
                 1 0 0 1 0 1 1 0 0 1 1 0 1 0 0 1]);

Walsh_Output = WALSH16_CODES(S2P_Output_dec + 1, :);

== matlab function HBC_PHY_Layer/PHYGenerator/PHYFrameConstructor ==
  data: PSDU input; PHYFrame output size=[1,9056]; PSDUdone input; section1 input; section1done input; selectRI input; done output
function [PHYFrame, done] = fcn(PSDU, PSDUdone,  section1, section1done, selectRI)
%#codegen
% Section 1 is maximum of 896 bits and PSDU is 8160 bits. Thus, PHYFrame is
% 9056 bits wide. 
PHYFrame = boolean(zeros(1,9056)); 
psdu = boolean(zeros(1,8160)); 
done = false;
psdu = transpose(PSDU); 
if(PSDUdone && section1done)
    if (selectRI) % Full Section1 is used to create frame
        PHYFrame = [section1, psdu]; 
        done = true; 
    else % only first 800 bits of Section1 is used to create frame
        PHYFrame = [section1(1:800), psdu, boolean(zeros(1,96))]; 
        done = true;    
    end 
end

== matlab function HBC_PHY_Layer/PHYGenerator/DataValidation ==
  data: dataIndx input; ValidData output; realData input; ValidIn input
function ValidData = fcn(dataIndx, realData, ValidIn)
%#codegen
ValidData = false; 
if (ValidIn) % Is the current sample a Valid piece of data from the serializer
    if(dataIndx <= realData) % Is the current sample within the value of the expected data
        ValidData = true; 
    else 
        ValidData = false; 
    end 
end

== matlab function HBC_PHY_Layer/MATLAB Function ==
  data: data input; DataIn output; numWalshCodes output
function [DataIn, numWalshCodes] = fcn(data)
%#codegen
numWalshCodes = ceil(length(data)/4);
temp = zeros(1,4*ceil(length(data)/4));
temp(1:length(data)) = data; 
DataIn = temp';
